simulink library "sixDoFDynamics6x6"  (R2018b)
settings: Solver=VariableStepAuto  StartTime=0.0  StopTime=10.0  RelTol=1e-3
undefined symbols (not defined in the file): vcl
libraries: dspmtrx3 x2, eulAng2RotMat_ul x1, eulDot x1
settings Model: Creator=jldanie5  LastModifiedBy=jldanie5

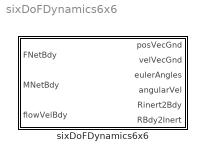
== system sixDoFDynamics6x6 ==
  sixDoFDynamics6x6 : Subsystem  VariantControl=(default)  mask{MMat=vcl.M6x6.Value, MaMat=vcl.Ma6x6.Value, DMat=vcl.D6x6.Value, rBtoCM=-vcl.RwingLE_cm.Value, initPos=vcl.initPosVecGnd.Value, initVel=vcl.initVelVecBdy.Value, initEulAngs=vcl.initEulAng.Value, initAngVel=vcl.initAngVelVec.Value}
      mask prompts: MMat "6x6 Mass Matrix"; MaMat "6x6 Added mass matrix"; DMat "6x6 Damping Matrix"; rBtoCM "Vector from Body Frame to CM"; initPos "Initial position"; initVel "Initial velocity"; initEulAngs "Initial Euler Angles"; initAngVel "Initial Angular Velocity Vec"
      mask init:
      | MtotMat = MMat + MaMat;
      | MinvMat = inv(MtotMat);

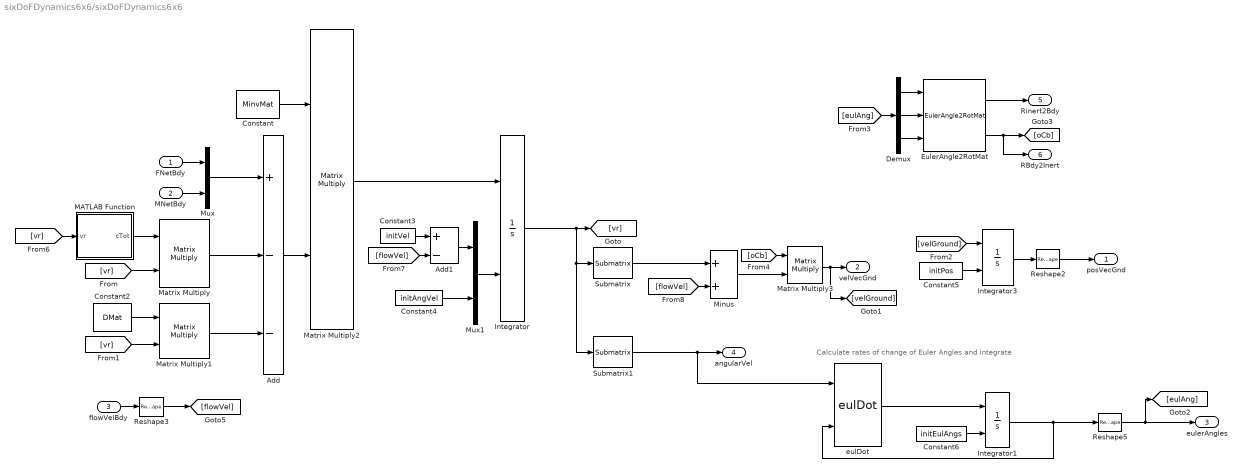
== system sixDoFDynamics6x6/sixDoFDynamics6x6 ==
  note: Calculate rates of change of Euler Angles and integrate
  FNetBdy : Inport
  MNetBdy : Inport  Port=2
  flowVelBdy : Inport  Port=3
  Add : Sum  Inputs=+--
  Add1 : Sum  Inputs=+-
  Constant : Constant  Value=MinvMat  VectorParams1D=off
  Constant2 : Constant  Value=DMat
  Constant3 : Constant  Value=initVel
  Constant4 : Constant  Value=initAngVel
  Constant5 : Constant  Value=initPos
  Constant6 : Constant  Value=initEulAngs
  Demux : Demux  Outputs=3
  EulerAngle2RotMat : eulAng2RotMat_ul/EulerAngle2RotMat  SystemSampleTime=-1
  Integrator : Integrator  InitialConditionSource=external
  Integrator1 : Integrator  InitialConditionSource=external  InitialCondition=initEulAngs
  Integrator3 : Integrator  InitialConditionSource=external  InitialCondition=initPos
  MATLAB Function : MATLAB Function  TreatAsAtomicUnit=on  mask{MMat=MMat, MaMat=MaMat, rBtoCM=rBtoCM}
      mask prompts: MMat "6x6 Mass Matrix"; MaMat "6x6 Added Mass Matrix"; rBtoCM "Vec From Body frame to CM"
  Matrix Multiply{,1..3} (4 alike) : Product  Multiplication=Matrix(*)
  Minus : Sum
  Mux : Mux  Inputs=2
  Mux1 : Mux  Inputs=2
  Reshape2 : Reshape  OutputDimensionality=Column vector (2-D)
  Reshape3 : Reshape  OutputDimensionality=Column vector (2-D)
  Reshape5 : Reshape  OutputDimensionality=Column vector (2-D)
  Submatrix : dspmtrx3/Submatrix  RowSpan=Range of rows  RowStartMode=First  RowStartIndex=1  RowEndMode=Index  RowEndIndex=3  ColSpan=All columns  ColStartMode=First  ColStartIndex=1  ColEndMode=Last  ColEndIndex=1
  Submatrix1 : dspmtrx3/Submatrix  RowSpan=Range of rows  RowStartMode=Index  RowStartIndex=4  RowEndMode=Last  RowEndIndex=1  ColSpan=All columns  ColStartMode=First  ColStartIndex=1  ColEndMode=Last  ColEndIndex=1
  eulDot : eulDot/eulDot  SystemSampleTime=-1
  posVecGnd : Outport
  velVecGnd : Outport  Port=2
  eulerAngles : Outport  Port=3
  angularVel : Outport  Port=4
  Rinert2Bdy : Outport  Port=5
  RBdy2Inert : Outport  Port=6
  wires:
  FNetBdy/1 -> Mux/1
  MNetBdy/1 -> Mux/2
  MATLAB Function/1(cTot) -> Matrix Multiply/1
  [vr] -> Matrix Multiply/2
  Constant2/1 -> Matrix Multiply1/1
  [vr] -> Matrix Multiply1/2
  Matrix Multiply1/1 -> Add/3
  Matrix Multiply/1 -> Add/2
  Mux/1 -> Add/1
  Add/1 -> Matrix Multiply2/2
  Constant/1 -> Matrix Multiply2/1
  Matrix Multiply2/1 -> Integrator/1
  Integrator/1 -> [vr], Submatrix1/1, Submatrix/1
  Constant4/1 -> Mux1/2
  Mux1/1 -> Integrator/2
  Integrator3/1 -> Reshape2/1
  Demux/3 -> EulerAngle2RotMat/3
  Demux/1 -> EulerAngle2RotMat/1
  EulerAngle2RotMat/2 -> RBdy2Inert/1, [oCb]
  Reshape2/1 -> posVecGnd/1
  Demux/2 -> EulerAngle2RotMat/2
  Constant5/1 -> Integrator3/2
  [eulAng] -> Demux/1
  eulDot/1 -> Integrator1/1
  Integrator1/1 -> eulDot/2, Reshape5/1
  Constant6/1 -> Integrator1/2
  Reshape5/1 -> eulerAngles/1, [eulAng]
  Submatrix1/1 -> eulDot/1, angularVel/1
  [vr] -> MATLAB Function/1(vr)
  flowVelBdy/1 -> Reshape3/1
  Reshape3/1 -> [flowVel]
  [flowVel] -> Minus/2
  [flowVel] -> Add1/2
  [velGround] -> Integrator3/1
  Constant3/1 -> Add1/1
  EulerAngle2RotMat/1 -> Rinert2Bdy/1
  Add1/1 -> Mux1/1
  Submatrix/1 -> Minus/1
  Minus/1 -> Matrix Multiply3/2
  [oCb] -> Matrix Multiply3/1
  Matrix Multiply3/1 -> [velGround], velVecGnd/1

== matlab function sixDoFDynamics6x6/MATLAB Function ==
  data: vr input; cTot output; MMat parameter; MaMat parameter; rBtoCM parameter
function cTot = fcn(vr, MMat, MaMat, rBtoCM)
    S=@(v) [0 -v(3) v(2);v(3) 0 -v(1);-v(2) v(1) 0];
    %Assume mass is located at (1,1) of the mass matrix
    m=MMat(1,1);
    %Assume intertia is located at bottom right 3x3 of the mass matrix
    I=MMat(4:6,4:6);
    %Renaming
    v1=vr(1:3);
    v2=vr(4:6);
    A11=MaMat(1:3,1:3);
    A12=MaMat(1:3,4:6);
    A21=MaMat(4:6,1:3);
    A22=MaMat(4:6,4:6);
    %Calulate Components, add, then return cTot
    crb=[m*S(v2) -m*S(v2)*S(rBtoCM);m*S(rBtoCM)*S(v2) -S(I*v2)];
    ca=[zeros(3) -S(A11*v1 + A12*v2);-S(A11*v1 + A12*v2) -S(A21*v1 + A22*v2)];
    cTot=crb+ca;
end
